simulink model "sampleModel1620"  (R2023a)
settings: Solver=VariableStepAuto  StartTime=0.0  StopTime=10.0  RelTol=1e-3
libraries: simulink x5, hdlsllib x4
settings Model: Creator=user1  LastModifiedBy=user1

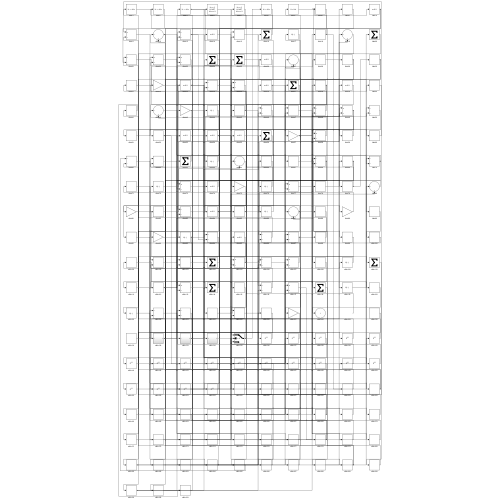
[thumbnail: Simulink's stored preview of the top-level diagram]
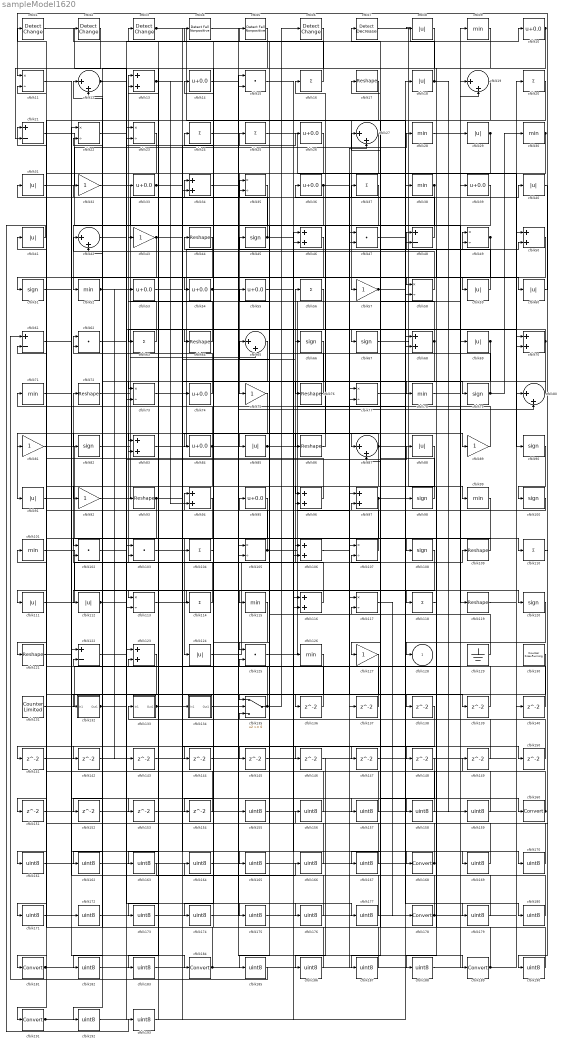
== system sampleModel1620 ==
  cfblk{1..3,6} (4 alike) : simulink/Logic and Bit Operations/Detect Change  vinit=0  OutDataTypeStr=boolean
      settings: LibrarySourceBlock=|
      | hdlsllib/Logic and Bit
      | Operations/Detect
      | Change
  cfblk{10,14,26,33,36,39,53..55,74,84,95} (12 alike) : Bias  Bias=0.0  SaturateOnIntegerOverflow=off
  cfblk{45,51,66..67,79,82,90,98,100,108,120} (11 alike) : Signum
  cfblk{9,28,30,38,52,71,78,99,101,115,126} (11 alike) : MinMax
  cfblk{15,47,62,102..103,125} (6 alike) : DotProduct  OutDataTypeStr=Inherit: Inherit via internal rule
  cfblk{16,20,24..25,37,56,63,104,110,114,118} (11 alike) : Sum  Inputs=+
  cfblk{11,22..23,35,49,58,73,77,105,107,113,117} (12 alike) : Product  Inputs=*/  RndMeth=Zero  SaturateOnIntegerOverflow=on
  cfblk{13,34,46,50,68,70,83,94,96..97,106,116,123} (13 alike) : Sum
  cfblk{17,44,64,72,76,86,93,109,119,121} (10 alike) : Reshape
  cfblk{8,18,29,31,40..41,59..60,69,85,88,91,111..112,124} (15 alike) : Abs  SaturateOnIntegerOverflow=off
  cfblk{12,19,27,42,65,80,87} (7 alike) : Sum  Inputs=|++
  cfblk{21,48,61,122} (4 alike) : Sum  Inputs=+-
  cfblk{32,43,57,75,81,89,92,127} (8 alike) : Gain
  cfblk129 : Ground
  cfblk130 : hdlsllib/Sources/Counter Free-Running  NumBits=16  tsamp=-1
  cfblk131 : hdlsllib/Sources/Counter Limited  uplimit=7  tsamp=-1
  cfblk132 : Subsystem
      settings: LibrarySourceBlock=|
      | hdlsllib/Ports &
      | Subsystems/Subsystem
  cfblk133 : Subsystem
      settings: LibrarySourceBlock=|
      | hdlsllib/Ports &
      | Subsystems/Subsystem
  cfblk134 : Subsystem
      settings: LibrarySourceBlock=|
      | hdlsllib/Ports &
      | Subsystems/Subsystem
  cfblk135 : Switch  SaturateOnIntegerOverflow=off  InputSameDT=off
  cfblk{136..154} (19 alike) : Delay  SampleTime=1
  cfblk{155..159,161..167,169..177,179..180,182..183,185..188,190,192..193} (32 alike) : DataTypeConversion  OutDataTypeStr=uint8  SaturateOnIntegerOverflow=off  RndMeth=Floor
  cfblk{160,168,178,181,184,189,191} (7 alike) : DataTypeConversion  SaturateOnIntegerOverflow=off  RndMeth=Floor
  cfblk4 : hdlsllib/Logic and Bit Operations/Detect Fall Nonpositive  vinit=0  OutDataTypeStr=boolean
  cfblk5 : hdlsllib/Logic and Bit Operations/Detect Fall Nonpositive  vinit=0  OutDataTypeStr=boolean
  cfblk7 : simulink/Logic and Bit Operations/Detect Decrease  vinit=0.0  OutDataTypeStr=boolean
      settings: LibrarySourceBlock=|
      | hdlsllib/Logic and Bit
      | Operations/Detect
      | Decrease
  cfblk128 : Outport  VectorParamsAs1DForOutWhenUnconnected=off
  wires:
  cfblk135/1 -> cfblk6/1, cfblk94/1
  cfblk7/1 -> cfblk79/1
  cfblk36/1 -> cfblk118/1, cfblk185/1
  cfblk28/1 -> cfblk29/1
  cfblk77/1 -> cfblk133/1(In1)
  cfblk90/1 -> cfblk100/1
  cfblk113/1 -> cfblk120/1
  cfblk124/1 -> cfblk56/1
  cfblk125/1 -> cfblk9/1
  cfblk86/1 -> cfblk36/1
  cfblk114/1 -> cfblk72/1
  cfblk111/1 -> cfblk109/1
  cfblk120/1 -> cfblk128/1
  cfblk116/1 -> cfblk13/1
  cfblk19/1 -> cfblk57/1
  cfblk132/1(Out1) -> cfblk25/1, cfblk10/1
  cfblk117/1 -> cfblk178/1
  cfblk33/1 -> cfblk146/1, cfblk147/1
  cfblk38/1 -> cfblk52/1, cfblk86/1
  cfblk52/1 -> cfblk67/1, cfblk143/1
  cfblk55/1 -> cfblk116/1
  cfblk105/1 -> cfblk62/1, cfblk27/2
  cfblk69/1 -> cfblk73/2, cfblk144/1
  cfblk68/1 -> cfblk112/1, cfblk17/1, cfblk85/1
  cfblk27/1 -> cfblk75/1
  cfblk58/1 -> cfblk42/1
  cfblk123/1 -> cfblk191/1
  cfblk31/1 -> cfblk28/1
  cfblk97/1 -> cfblk132/1(In1), cfblk179/1
  cfblk18/1 -> cfblk8/1, cfblk159/1
  cfblk79/1 -> cfblk35/1, cfblk30/1
  cfblk67/1 -> cfblk99/1
  cfblk87/1 -> cfblk96/1, cfblk49/2, cfblk83/1
  cfblk129/1 -> cfblk55/1
  cfblk96/1 -> cfblk21/1
  cfblk21/1 -> cfblk119/1
  cfblk60/1 -> cfblk11/1
  cfblk98/1 -> cfblk37/1
  cfblk59/1 -> cfblk7/1
  cfblk81/1 -> cfblk110/1
  cfblk92/1 -> cfblk40/1
  cfblk46/1 -> cfblk181/1
  cfblk61/1 -> cfblk184/1
  cfblk9/1 -> cfblk12/2
  cfblk74/1 -> cfblk32/1
  cfblk75/1 -> cfblk91/1
  cfblk94/1 -> cfblk124/1
  cfblk49/1 -> cfblk76/1, cfblk68/2
  cfblk45/1 -> cfblk31/1, cfblk50/2
  cfblk25/1 -> cfblk90/1
  cfblk131/1 -> cfblk19/1
  cfblk101/1 -> cfblk115/1
  cfblk64/1 -> cfblk3/1
  cfblk99/1 -> cfblk113/1
  cfblk65/1 -> cfblk105/2
  cfblk95/1 -> cfblk111/1
  cfblk30/1 -> cfblk51/1, cfblk64/1
  cfblk109/1 -> cfblk108/1
  cfblk71/1 -> cfblk168/1
  cfblk1/1 -> cfblk23/2
  cfblk2/1 -> cfblk21/2
  cfblk23/1 -> cfblk82/1
  cfblk70/1 -> cfblk92/1, cfblk63/1
  cfblk39/1 -> cfblk127/1
  cfblk3/1 -> cfblk98/1, cfblk87/1
  cfblk66/1 -> cfblk102/1
  cfblk17/1 -> cfblk81/1
  cfblk78/1 -> cfblk39/1
  cfblk47/1 -> cfblk160/1
  cfblk63/1 -> cfblk43/1
  cfblk93/1 -> cfblk113/2, cfblk66/1
  cfblk133/1(Out1) -> cfblk134/1(In1), cfblk26/1
  cfblk56/1 -> cfblk125/1
  cfblk48/1 -> cfblk16/1
  cfblk83/1 -> cfblk48/1
  cfblk107/1 -> cfblk41/1
  cfblk112/1 -> cfblk88/1, cfblk106/1
  cfblk104/1 -> cfblk34/1
  cfblk82/1 -> cfblk65/2
  cfblk12/1 -> cfblk42/2, cfblk70/2
  cfblk32/1 -> cfblk104/1
  cfblk10/1 -> cfblk58/1, cfblk54/1
  cfblk89/1 -> cfblk14/1
  cfblk43/1 -> cfblk78/1, cfblk151/1
  cfblk76/1 -> cfblk35/2
  cfblk37/1 -> cfblk135/1
  cfblk57/1 -> cfblk49/1, cfblk180/1
  cfblk119/1 -> cfblk80/1
  cfblk54/1 -> cfblk89/1, cfblk150/1
  cfblk13/1 -> cfblk74/1, cfblk94/2
  cfblk102/1 -> cfblk53/1
  cfblk16/1 -> cfblk2/1
  cfblk29/1 -> cfblk77/2, cfblk87/2
  cfblk85/1 -> cfblk38/1, cfblk5/1
  cfblk24/1 -> cfblk189/1
  cfblk72/1 -> cfblk19/2
  cfblk34/1 -> cfblk59/1
  cfblk80/1 -> cfblk73/1
  cfblk100/1 -> cfblk96/2
  cfblk51/1 -> cfblk60/1
  cfblk84/1 -> cfblk121/1, cfblk11/2, cfblk80/2, cfblk158/1
  cfblk8/1 -> cfblk84/1
  cfblk62/1 -> cfblk136/1
  cfblk136/1 -> cfblk1/1
  cfblk137/1 -> cfblk65/1
  cfblk106/1 -> cfblk138/1
  cfblk11/1 -> cfblk139/1
  cfblk139/1 -> cfblk13/2
  cfblk140/1 -> cfblk23/1
  cfblk88/1 -> cfblk141/1
  cfblk141/1 -> cfblk70/1
  cfblk108/1 -> cfblk142/1
  cfblk142/1 -> cfblk12/1
  cfblk143/1 -> cfblk107/1
  cfblk144/1 -> cfblk97/1
  cfblk73/1 -> cfblk145/1
  cfblk145/1 -> cfblk77/1
  cfblk147/1 -> cfblk27/1
  cfblk53/1 -> cfblk148/1
  cfblk149/1 -> cfblk135/2
  cfblk150/1 -> cfblk125/2
  cfblk151/1 -> cfblk34/2
  cfblk26/1 -> cfblk152/1
  cfblk152/1 -> cfblk105/1
  cfblk121/1 -> cfblk153/1
  cfblk153/1 -> cfblk50/1
  cfblk115/1 -> cfblk154/1
  cfblk154/1 -> cfblk101/1
  cfblk4/1 -> cfblk155/1
  cfblk155/1 -> cfblk95/1
  cfblk110/1 -> cfblk156/1
  cfblk156/1 -> cfblk4/1
  cfblk22/1 -> cfblk157/1
  cfblk157/1 -> cfblk93/1
  cfblk158/1 -> cfblk22/1
  cfblk159/1 -> cfblk22/2
  cfblk160/1 -> cfblk149/1, cfblk102/2
  cfblk127/1 -> cfblk161/1
  cfblk161/1 -> cfblk47/1
  cfblk5/1 -> cfblk162/1
  cfblk162/1 -> cfblk47/2
  cfblk126/1 -> cfblk163/1
  cfblk164/1 -> cfblk126/1
  cfblk103/1 -> cfblk165/1
  cfblk165/1 -> cfblk68/1
  cfblk163/1 -> cfblk166/1
  cfblk166/1 -> cfblk103/1
  cfblk148/1 -> cfblk167/1
  cfblk167/1 -> cfblk103/2
  cfblk168/1 -> cfblk135/3, cfblk107/2
  cfblk134/1(Out1) -> cfblk169/1
  cfblk169/1 -> cfblk71/1
  cfblk15/1 -> cfblk170/1
  cfblk170/1 -> cfblk45/1
  cfblk138/1 -> cfblk171/1
  cfblk171/1 -> cfblk15/1
  cfblk91/1 -> cfblk172/1
  cfblk172/1 -> cfblk15/2
  cfblk44/1 -> cfblk173/1
  cfblk173/1 -> cfblk18/1
  cfblk50/1 -> cfblk174/1
  cfblk174/1 -> cfblk44/1
  cfblk122/1 -> cfblk175/1
  cfblk175/1 -> cfblk140/1
  cfblk14/1 -> cfblk176/1
  cfblk176/1 -> cfblk122/1
  cfblk42/1 -> cfblk177/1
  cfblk177/1 -> cfblk122/2
  cfblk178/1 -> cfblk164/1, cfblk83/2
  cfblk179/1 -> cfblk117/1
  cfblk180/1 -> cfblk117/2
  cfblk181/1 -> cfblk137/1, cfblk106/2
  cfblk35/1 -> cfblk182/1
  cfblk182/1 -> cfblk46/1
  cfblk6/1 -> cfblk183/1
  cfblk183/1 -> cfblk46/2
  cfblk184/1 -> cfblk33/1, cfblk69/1
  cfblk185/1 -> cfblk61/1
  cfblk146/1 -> cfblk186/1
  cfblk186/1 -> cfblk61/2
  cfblk20/1 -> cfblk187/1
  cfblk187/1 -> cfblk62/2
  cfblk118/1 -> cfblk188/1
  cfblk188/1 -> cfblk20/1
  cfblk189/1 -> cfblk48/2, cfblk97/2
  cfblk40/1 -> cfblk190/1
  cfblk190/1 -> cfblk24/1
  cfblk191/1 -> cfblk58/2, cfblk114/1, cfblk116/2
  cfblk130/1 -> cfblk192/1
  cfblk192/1 -> cfblk123/1
  cfblk41/1 -> cfblk193/1
  cfblk193/1 -> cfblk123/2

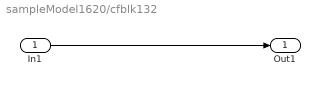
== system sampleModel1620/cfblk132 ==
  In1 : Inport
  Out1 : Outport
  wires:
  In1/1 -> Out1/1

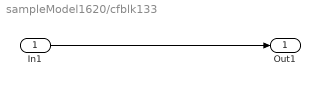
== system sampleModel1620/cfblk133 ==
  In1 : Inport
  Out1 : Outport
  wires:
  In1/1 -> Out1/1

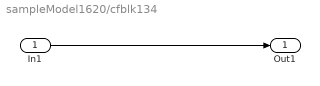
== system sampleModel1620/cfblk134 ==
  In1 : Inport
  Out1 : Outport
  wires:
  In1/1 -> Out1/1
